simulink model "Spatial4barDyn"  (Simulink 8.6)
settings: Solver=ode45  StartTime=0.0  StopTime=10  MaxStep=.01  RelTol=1e-3
model workspace: external: MAT-File C:\Users\John\Dropbox\phd\MsimSimulations\Msim\MotionSim\simulink\Spatial4barDyn-SIMULINKPARAM.mat (data not in the file)
values from neighbouring files (symbols this model uses):
  sysmodel =     [AUTO2-SIMULINKPARAM.mat]    (also in AUTO4-SIMULINKPARAM.mat; Chapter7Dyn2dCrankRocker-SIMULINKPARAM.mat; Spatial4barDyn-SIMULINKPARAM.mat)
undefined symbols (not defined in the file or in its folder): selectnum
libraries: simulink x1
settings Model: Creator=JohnD  LastModifiedBy=John  ExtModeTrigDuration=100
settings OptimizationCC: OptimizeModelRefInitCode=on  LifeSpan=1
settings DebuggingCC: SolverPrmCheckMsg=none  FcnCallInpInsideContextMsg=EnableAllAsWarning  StrictBusMsg=Warning
settings HardwareCC: ProdLargestAtomicInteger=Long  ProdLargestAtomicFloat=Double  ProdEndianess=LittleEndian  ProdHWDeviceType=ARM Compatible->ARM Cortex
settings RTWCC: SystemTargetFile=realtime.tlc  GenerateMakefile=off  TemplateMakefile=realtime.tmf  Description=Real-Time Toolbox  RTWVerbose=off
settings CodeAppCC: CustomSymbolStrType=$N$R$M  InternalIdentifier=Classic
settings STFCustomTargetCC: TargetLibSuffix=.a  GenerateSampleERTMain=on  ERTCustomFileBanners=on  SupportNonInlinedSFcns=off  SupportVariableSizeSignals=on  MATLABClassNameForMDSCustomization=Simulink.SoftwareTarget.ERTCustomization  GRTInterface=off  SystemTargetFile=realtime.tlc
settings ERTTargetCC: MultiwordLength=2048  GenerateSampleERTMain=on  ParMdlRefBuildCompliant=off  CompOptLevelCompliant=off  ConcurrentExecutionCompliant=off  CombineOutputUpdateFcns=off  ERTFirstTimeCompliant=off  SupportContinuousTime=on  SupportVariableSizeSignals=on  ModelStepFunctionPrototypeControlCompliant=off  CPPClassGenCompliant=off  UseToolchainInfoCompliant=off  ExtModeMexFile=noextcomm  ExtModeMexArgs='10.10.10.1' 0 17725  ERTSrcFileBannerTemplate=realtime_code_template.cgt  ERTHdrFileBannerTemplate=realtime_code_template.cgt  ERTDataSrcFileTemplate=realtime_code_template.cgt  ERTDataHdrFileTemplate=realtime_code_template.cgt  ERTCustomFileTemplate=realtime_file_process.tlc  ConvertIfToSwitch=off  SuppressUnreachableDefaultCases=off
settings SettingsController: Description=Run on Hardware Dialog  TargetExtensionPlatform=None

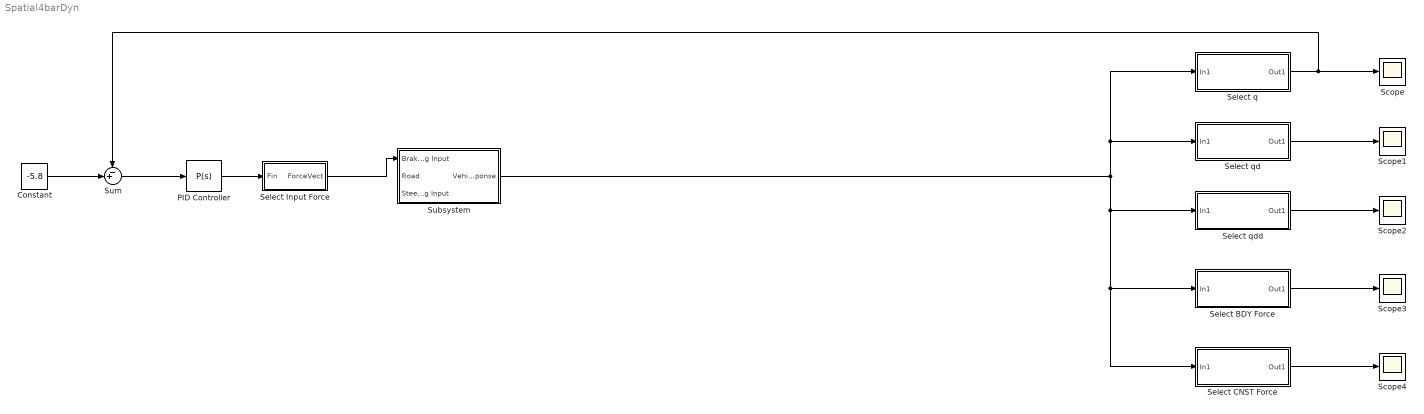
== system Spatial4barDyn ==
  Constant : Constant  Value=-5.8
  PID Controller : simulink/Continuous/PID Controller  Controller=P  TimeDomain=Continuous-time  SampleTime=-1  IntegratorMethod=Forward Euler  FilterMethod=Forward Euler  Form=Parallel  UseFilter=on  ControllerParametersSource=internal  P=-100  I=4.25362009082164e-006  D=3020499.89949622  N=0.0109577188347424  InitialConditionSource=internal  InitialConditionForIntegrator=0  InitialConditionForFilter=0  ExternalReset=none  LimitOutput=off  UpperSaturationLimit=inf  LowerSaturationLimit=-inf  LinearizeAsGain=off  AntiWindupMode=none  Kb=1  TrackingMode=off  Kt=1  PParamMin=[]  PParamMax=[]  IParamMin=[]  IParamMax=[]  DParamMin=[]  DParamMax=[]  NParamMin=[]  NParamMax=[]  KbParamMin=[]  KbParamMax=[]  KtParamMin=[]  KtParamMax=[]  POutMin=[]  POutMax=[]  IOutMin=[]  IOutMax=[]  DOutMin=[]  DOutMax=[]  NOutMin=[]  NOutMax=[]  KbOutMin=[]  KbOutMax=[]  KtOutMin=[]  KtOutMax=[]  IntegratorOutMin=[]  IntegratorOutMax=[]  FilterOutMin=[]  FilterOutMax=[]  SumOutMin=[]  SumOutMax=[]  SumI1OutMin=[]  SumI1OutMax=[]  SumI2OutMin=[]  SumI2OutMax=[]  SumI3OutMin=[]  SumI3OutMax=[]  SumDOutMin=[]  SumDOutMax=[]  SaturationOutMin=[]  SaturationOutMax=[]  IntegratorContinuousStateAttributes=''  IntegratorStateMustResolveToSignalObject=off  IntegratorRTWStateStorageClass=Auto  FilterContinuousStateAttributes=''  FilterStateMustResolveToSignalObject=off  FilterRTWStateStorageClass=Auto  DifferentiatorICPrevScaledInput=0  DifferentiatorOutMin=[]  DifferentiatorOutMax=[]
  Scope{,1..4} (5 alike) : Scope
  Select BDY Force : Subsystem  mask{Bodynum=3, Selectnum=Tx}
      mask prompts: Bodynum "Body Number"; Selectnum "Select Coordinate"
      mask TypeOptions Selectnum: Fx | Fy | Fz | Tx | Ty | Tz
      mask Display:
      | port_label('input',1,'Coord');
      | port_label('output',1,'BDY Force');
  Select CNST Force : Subsystem  mask{Bodynum=1, Selectnum=Tx}
      mask prompts: Bodynum "Body Number"; Selectnum "Select Coordinate"
      mask TypeOptions Selectnum: Fx | Fy | Fz | Tx | Ty | Tz
      mask Display:
      | port_label('input',1,'Coord');
      | port_label('output',1,'CNST Force');
  Select Input Force : Subsystem  mask{BodyNum=1, ForceNum=Tx}
      mask prompts: BodyNum "Body Number"; ForceNum "Force"
      mask TypeOptions ForceNum: Fx | Fy | Fz | Tx | Ty | Tz
  Select q : Subsystem  mask{Bodynum=3, Selectnum=X}
      mask prompts: Bodynum "Body Number"; Selectnum "Select Coordinate"
      mask TypeOptions Selectnum: X | Y | Z | e0 | e1 | e2 | e3
      mask Display:
      | port_label('input',1,'Coord');
      | port_label('output',1,'q');
  Select qd : Subsystem  mask{Bodynum=3, Selectnum=Xd}
      mask prompts: Bodynum "Body Number"; Selectnum "Select Coordinate"
      mask TypeOptions Selectnum: Xd | Yd | Zd | e0d | e1d | e2d | e3d
      mask Display:
      | port_label('input',1,'Coord');
      | port_label('output',1,'qd');
  Select qdd : Subsystem  mask{Bodynum=3, Selectnum=Xdd}
      mask prompts: Bodynum "Body Number"; Selectnum "Select Coordinate"
      mask TypeOptions Selectnum: Xdd | Ydd | Zdd | e0dd | e1dd | e2dd | e3dd
      mask Display:
      | port_label('input',1,'Coord');
      | port_label('output',1,'qdd');
  Subsystem : Subsystem
  Sum : Sum  Inputs=-+|
  wires:
  PID Controller/1 -> Select Input Force/1(Fin)
  Select q/1(Out1) -> Scope/1, Sum/1
  Select qd/1(Out1) -> Scope1/1
  Sum/1 -> PID Controller/1
  Constant/1 -> Sum/2
  Select qdd/1(Out1) -> Scope2/1
  Select BDY Force/1(Out1) -> Scope3/1
  Select CNST Force/1(Out1) -> Scope4/1
  Subsystem/1(Vehicle Response) -> Select qdd/1(In1), Select BDY Force/1(In1), Select CNST Force/1(In1), Select q/1(In1), Select qd/1(In1)
  Select Input Force/1(ForceVect) -> Subsystem/1(Braking Input)

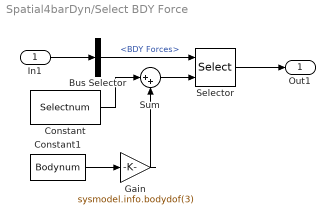
== system Spatial4barDyn/Select BDY Force ==
  In1 : Inport
  Bus Selector : BusSelector  OutputSignals=BDY Forces
  Constant : Constant  Value=Selectnum
  Constant1 : Constant  Value=Bodynum
  Gain : Gain  Gain=sysmodel.info.bodydof(3)
  Selector : Selector  InputPortWidth=sysmodel.info.bodies*sysmodel.info.bodydof(3)  IndexOptions=Index vector (port)  Indices=[Bodynum+selectnum]  OutputSizes=1
  Sum : Sum  Inputs=|++
  Out1 : Outport
  wires:
  Selector/1 -> Out1/1
  Constant1/1 -> Gain/1
  Sum/1 -> Selector/2
  Constant/1 -> Sum/1
  Gain/1 -> Sum/2
  In1/1 -> Bus Selector/1
  Bus Selector/1 -> Selector/1  "<BDY Forces>"

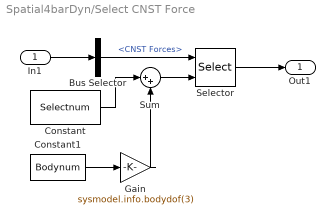
== system Spatial4barDyn/Select CNST Force ==
  In1 : Inport
  Bus Selector : BusSelector  OutputSignals=CNST Forces
  Constant : Constant  Value=Selectnum
  Constant1 : Constant  Value=Bodynum
  Gain : Gain  Gain=sysmodel.info.bodydof(3)
  Selector : Selector  InputPortWidth=sysmodel.info.bodies*sysmodel.info.bodydof(3)  IndexOptions=Index vector (port)  Indices=[Bodynum+selectnum]  OutputSizes=1
  Sum : Sum  Inputs=|++
  Out1 : Outport
  wires:
  Selector/1 -> Out1/1
  Constant1/1 -> Gain/1
  Sum/1 -> Selector/2
  Constant/1 -> Sum/1
  Gain/1 -> Sum/2
  In1/1 -> Bus Selector/1
  Bus Selector/1 -> Selector/1  "<CNST Forces>"

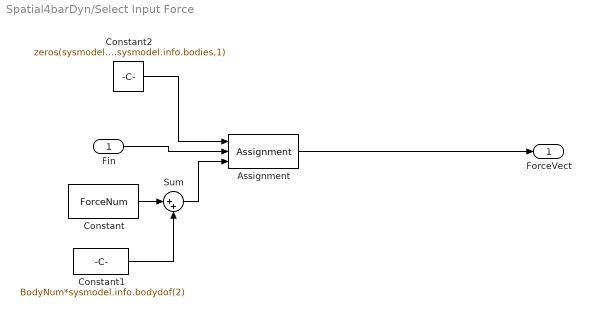
== system Spatial4barDyn/Select Input Force ==
  Fin : Inport
  Assignment : Assignment  IndexOptions=Index vector (port)  Indices=9  OutputSizes=1
  Constant : Constant  Value=ForceNum
  Constant1 : Constant  Value=BodyNum*sysmodel.info.bodydof(2)
  Constant2 : Constant  Value=zeros(sysmodel.info.bodydof(2)*sysmodel.info.bodies,1)
  Sum : Sum  Inputs=|++
  ForceVect : Outport
  wires:
  Assignment/1 -> ForceVect/1
  Constant2/1 -> Assignment/1
  Fin/1 -> Assignment/2
  Constant1/1 -> Sum/2
  Constant/1 -> Sum/1
  Sum/1 -> Assignment/3

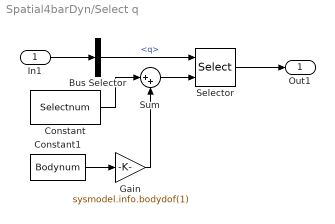
== system Spatial4barDyn/Select q ==
  In1 : Inport
  Bus Selector : BusSelector  OutputSignals=q
  Constant : Constant  Value=Selectnum
  Constant1 : Constant  Value=Bodynum
  Gain : Gain  Gain=sysmodel.info.bodydof(1)
  Selector : Selector  InputPortWidth=sysmodel.info.bodies*sysmodel.info.bodydof(1)  IndexOptions=Index vector (port)  Indices=[Bodynum+selectnum]  OutputSizes=1
  Sum : Sum  Inputs=|++
  Out1 : Outport
  wires:
  Selector/1 -> Out1/1
  Constant1/1 -> Gain/1
  Sum/1 -> Selector/2
  Constant/1 -> Sum/1
  Gain/1 -> Sum/2
  In1/1 -> Bus Selector/1
  Bus Selector/1 -> Selector/1  "<q>"

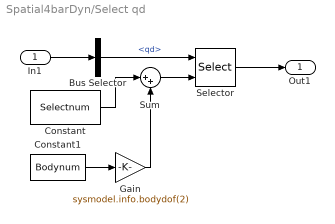
== system Spatial4barDyn/Select qd ==
  In1 : Inport
  Bus Selector : BusSelector  OutputSignals=qd
  Constant : Constant  Value=Selectnum
  Constant1 : Constant  Value=Bodynum
  Gain : Gain  Gain=sysmodel.info.bodydof(2)
  Selector : Selector  InputPortWidth=sysmodel.info.bodies*sysmodel.info.bodydof(2)  IndexOptions=Index vector (port)  Indices=[Bodynum+selectnum]  OutputSizes=1
  Sum : Sum  Inputs=|++
  Out1 : Outport
  wires:
  Selector/1 -> Out1/1
  Constant1/1 -> Gain/1
  Sum/1 -> Selector/2
  Constant/1 -> Sum/1
  Gain/1 -> Sum/2
  In1/1 -> Bus Selector/1
  Bus Selector/1 -> Selector/1  "<qd>"

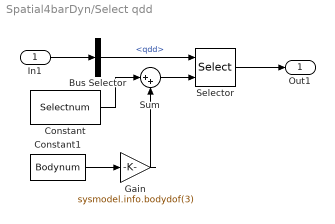
== system Spatial4barDyn/Select qdd ==
  In1 : Inport
  Bus Selector : BusSelector  OutputSignals=qdd
  Constant : Constant  Value=Selectnum
  Constant1 : Constant  Value=Bodynum
  Gain : Gain  Gain=sysmodel.info.bodydof(3)
  Selector : Selector  InputPortWidth=sysmodel.info.bodies*sysmodel.info.bodydof(3)  IndexOptions=Index vector (port)  Indices=[Bodynum+selectnum]  OutputSizes=1
  Sum : Sum  Inputs=|++
  Out1 : Outport
  wires:
  Selector/1 -> Out1/1
  Constant1/1 -> Gain/1
  Sum/1 -> Selector/2
  Constant/1 -> Sum/1
  Gain/1 -> Sum/2
  In1/1 -> Bus Selector/1
  Bus Selector/1 -> Selector/1  "<qdd>"

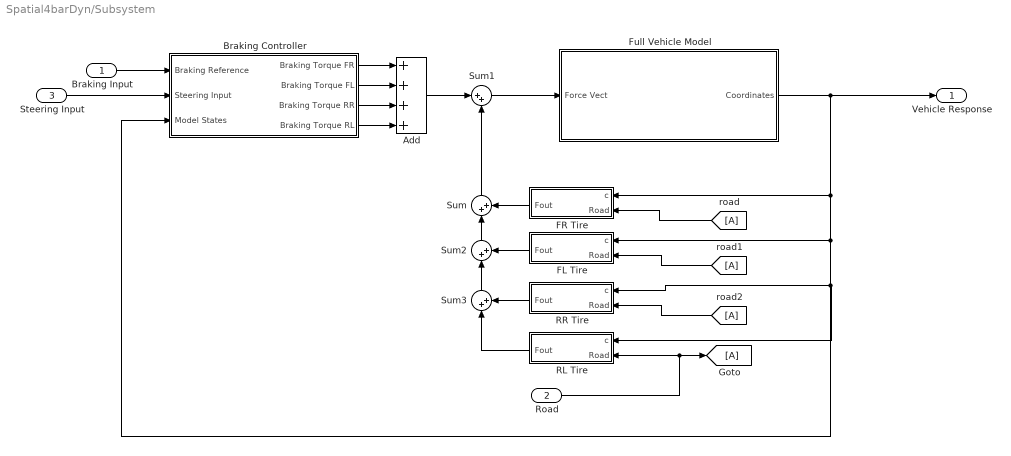
== system Spatial4barDyn/Subsystem ==
  Braking Input : Inport
  Road : Inport  Port=2
  Steering Input : Inport  Port=3
  Add : Sum  Inputs=++++
  Braking Controller : Subsystem
  FL Tire : Subsystem
  FR Tire : Subsystem
  Full Vehicle Model : Subsystem
  RL Tire : Subsystem
  RR Tire : Subsystem
  Sum{,1..3} (4 alike) : Sum  Inputs=|++
  Vehicle Response : Outport
  wires:
  Full Vehicle Model/1(Coordinates) -> Vehicle Response/1, Braking Controller/3(Model States), RL Tire/1(c), RR Tire/1(c), FL Tire/1(c), FR Tire/1(c)
  Sum/1 -> Sum1/2
  Sum1/1 -> Full Vehicle Model/1(Force Vect)
  FR Tire/1(Fout) -> Sum/2
  FL Tire/1(Fout) -> Sum2/2
  RR Tire/1(Fout) -> Sum3/2
  Sum2/1 -> Sum/1
  Sum3/1 -> Sum2/1
  RL Tire/1(Fout) -> Sum3/1
  [A] -> FR Tire/2(Road)
  [A] -> FL Tire/2(Road)
  [A] -> RR Tire/2(Road)
  Road/1 -> RL Tire/2(Road), [A]
  Braking Controller/1(Braking Torque FR) -> Add/1
  Braking Controller/2(Braking Torque FL) -> Add/2
  Braking Controller/3(Braking Torque RR) -> Add/3
  Braking Controller/4(Braking Torque RL) -> Add/4
  Add/1 -> Sum1/1
  Braking Input/1 -> Braking Controller/1(Braking Reference)
  Steering Input/1 -> Braking Controller/2(Steering Input)

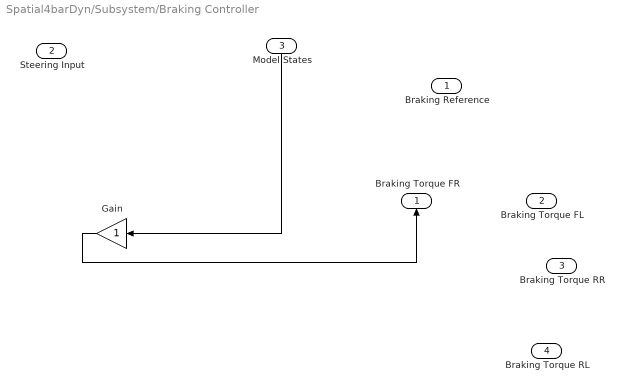
== system Spatial4barDyn/Subsystem/Braking Controller ==
  Braking Reference : Inport
  Steering Input : Inport  Port=2
  Model States : Inport  Port=3
  Gain : Gain
  Braking Torque FR : Outport
  Braking Torque FL : Outport  Port=2
  Braking Torque RR : Outport  Port=3
  Braking Torque RL : Outport  Port=4
  wires:
  Model States/1 -> Gain/1
  Gain/1 -> Braking Torque FR/1

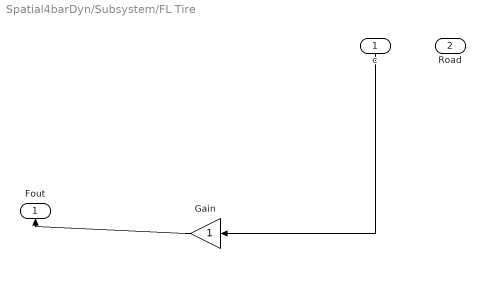
== system Spatial4barDyn/Subsystem/FL Tire ==
  c : Inport
  Road : Inport  Port=2
  Gain : Gain
  Fout : Outport
  wires:
  c/1 -> Gain/1
  Gain/1 -> Fout/1

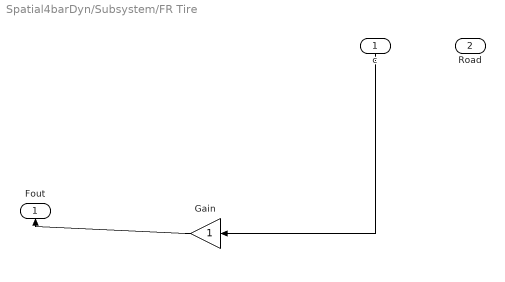
== system Spatial4barDyn/Subsystem/FR Tire ==
  c : Inport
  Road : Inport  Port=2
  Gain : Gain
  Fout : Outport
  wires:
  c/1 -> Gain/1
  Gain/1 -> Fout/1

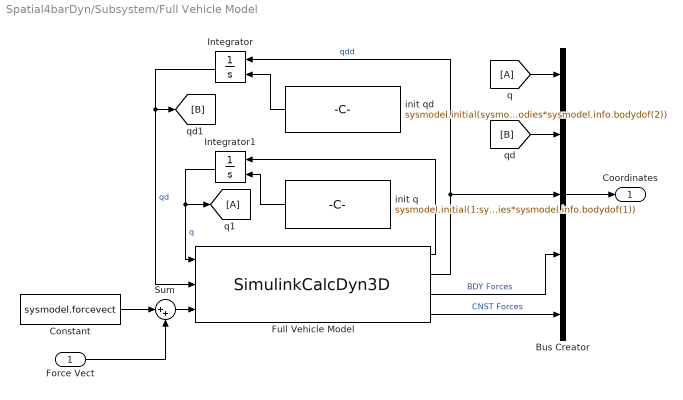
== system Spatial4barDyn/Subsystem/Full Vehicle Model ==
  Force Vect : Inport
  Bus Creator : BusCreator  Inputs=5
  Constant : Constant  Value=sysmodel.forcevect
  Full Vehicle Model : M-S-Function  FunctionName=SimulinkCalcDyn3D  Parameters=sysmodel
      mask Display:
      | image('mbs4.PNG');
      | port_label('output',1,'qd');
      | port_label('output',2,'qdd');
      | port_label('output',3,'Body Forces');
      | port_label('output',4,'Constraint Forces');
      | 
      | port_label('input',1,'q');
      | port_label('input',2,'qd');
  Integrator : Integrator  InitialConditionSource=external
  Integrator1 : Integrator  InitialConditionSource=external
  Sum : Sum  Inputs=|++
  init q : Constant  Value=sysmodel.initial(1:sysmodel.info.bodies*sysmodel.info.bodydof(1))
  init qd : Constant  Value=sysmodel.initial(sysmodel.info.bodies*sysmodel.info.bodydof(1)+1:sysmodel.info.bodies*sysmodel.info.bodydof(1)+sysmodel.info.bodies*sysmodel.info.bodydof(2))
  Coordinates : Outport
  wires:
  Integrator1/1 -> Full Vehicle Model/1, [A]  "q"
  Integrator/1 -> Full Vehicle Model/2, [B]  "qd"
  Full Vehicle Model/1 -> Integrator1/1
  Full Vehicle Model/2 -> Integrator/1, Bus Creator/3  "qdd"
  init q/1 -> Integrator1/2
  init qd/1 -> Integrator/2
  Full Vehicle Model/3 -> Bus Creator/4  "BDY Forces"
  Full Vehicle Model/4 -> Bus Creator/5  "CNST Forces"
  Sum/1 -> Full Vehicle Model/3
  Force Vect/1 -> Sum/2
  Constant/1 -> Sum/1
  [B] -> Bus Creator/2
  [A] -> Bus Creator/1
  Bus Creator/1 -> Coordinates/1

== system Spatial4barDyn/Subsystem/RL Tire ==
  c : Inport
  Road : Inport  Port=2
  Gain : Gain
  Fout : Outport
  wires:
  c/1 -> Gain/1
  Gain/1 -> Fout/1

== system Spatial4barDyn/Subsystem/RR Tire ==
  c : Inport
  Road : Inport  Port=2
  Gain : Gain
  Fout : Outport
  wires:
  c/1 -> Gain/1
  Gain/1 -> Fout/1
